simulink model "QuarterCarModel2"  (R2023b)
settings: Solver=VariableStepAuto  StartTime=0.0  StopTime=10.0  RelTol=1e-3
values from neighbouring files (symbols this model uses):
  d = 50    [QuarterCarWrapperScript.m]
  h_s = 1    [QuarterCarWrapperScript.m]
  h_u = 0.5    [QuarterCarWrapperScript.m]
  k_s = 50000    [QuarterCarWrapperScript.m]
  m_s = 50    [QuarterCarWrapperScript.m]
  m_t = 4    [QuarterCarWrapperScript.m]
settings Model: Creator=emily  LastModifiedBy=emily

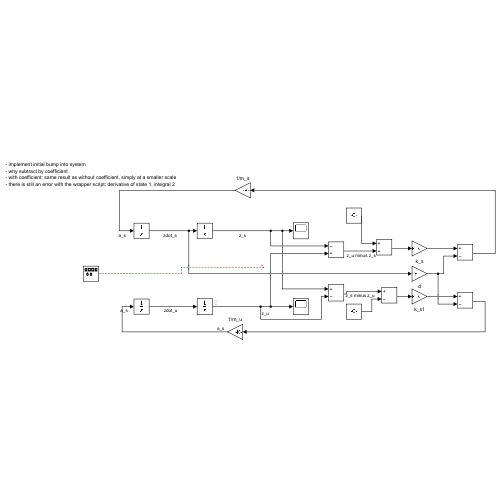
[thumbnail: Simulink's stored preview of the top-level diagram]
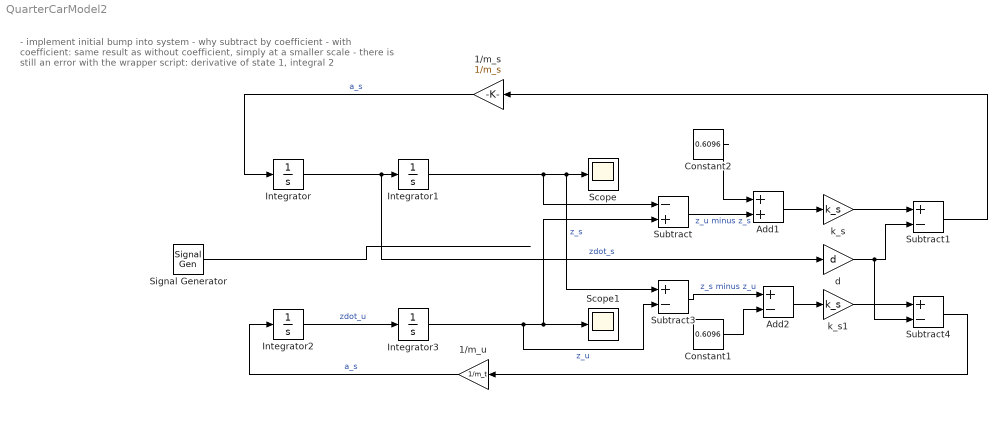
== system QuarterCarModel2 ==
  note: - implement initial bump into system
      | - why subtract by coefficient
      | - with coefficient: same result as without coefficient, simply at a smaller scale
      | - there is still an error with the wrapper script: derivative of state 1, integral 2
  1/m_s : Gain  Gain=1/m_s
  1/m_u : Gain  Gain=1/m_t
  Add1 : Sum
  Add2 : Sum  Inputs=+-
  Constant1 : Constant  Value=0.6096
  Constant2 : Constant  Value=0.6096
  Integrator : Integrator
  Integrator1 : Integrator  InitialCondition=h_s
  Integrator2 : Integrator
  Integrator3 : Integrator  InitialCondition=h_u
  Scope : Scope
  Scope1 : Scope
  Signal Generator : SignalGenerator  Amplitude=0.3  Frequency=3  Units=rad/sec
  Subtract : Sum  Inputs=-+
  Subtract1 : Sum  Inputs=+-
  Subtract3 : Sum  Inputs=+-
  Subtract4 : Sum  Inputs=+-
  d : Gain  Gain=d
  k_s : Gain  Gain=k_s
  k_s1 : Gain  Gain=k_s
  wires:
  1/m_s/1 -> Integrator/1  "a_s"
  Integrator2/1 -> Integrator3/1  "zdot_u"
  Subtract4/1 -> 1/m_u/1
  Constant1/1 -> Add2/2
  k_s1/1 -> Subtract4/1
  Subtract/1 -> Add1/2  "z_u minus z_s"
  1/m_u/1 -> Integrator2/1  "a_s"
  Constant2/1 -> Add1/1
  Integrator/1 -> d/1, Integrator1/1  "zdot_s"
  Add2/1 -> k_s1/1
  Subtract1/1 -> 1/m_s/1
  Subtract3/1 -> Add2/1  "z_s minus z_u"
  Add1/1 -> k_s/1
  k_s/1 -> Subtract1/1
  Integrator3/1 -> Subtract3/2, Subtract/2, Scope1/1  "z_u"
  Integrator1/1 -> Subtract3/1, Scope/1, Subtract/1  "z_s"
  d/1 -> Subtract4/2, Subtract1/2
  Signal Generator/1 -> ?
